simulink model "ev3_final"  (R2018b)
settings: Solver=FixedStepAuto  StartTime=0.0  StopTime=10.0  RelTol=1e-3  EnableMultiTasking=on
libraries: legoev3lib x9, dspstat3 x2
settings Model: ExtModeTrigDuration=2  Creator=chpark  LastModifiedBy=chpark
settings SolverCC: PositivePriorityOrder=on
settings OptimizationCC: EnhancedBackFolding=on  PassReuseOutputArgsAs=Individual arguments  MaxStackSize=64  OptimizeBlockOrder=speed  DifferentSizesBufferReuse=on  OptimizationCustomize=off
settings DebuggingCC: ParameterTunabilityLossMsg=error
settings HardwareCC: ProdBitPerPointer=32  ProdBitPerSizeT=32  ProdBitPerPtrDiffT=32  ProdLargestAtomicInteger=Long  ProdWordSize=32  ProdHWDeviceType=ARM Compatible->ARM 9  UseEmbeddedCoderFeatures=off  UseSimulinkCoderFeatures=off
settings SFSimCC: MATLABDynamicMemAlloc=off
settings RTWCC: SystemTargetFile=ert.tlc  HardwareBoard=LEGO MINDSTORMS EV3  TLCOptions="-aInlineSetEventsForThisBaseRateFcn=TLC_FALSE -aSuppressMultiTaskScheduler=TLC_FALSE  -aRateBasedStepFcn=0"  TemplateMakefile=ert_default_tmf  GenerateReport=on  Toolchain=Sourcery G++ Lite v2009q3  IncludeHyperlinkInReport=on  LaunchReport=on  GenerateTraceInfo=on  GenerateTraceReport=on  GenerateTraceReportSl=on  GenerateTraceReportSf=on  GenerateTraceReportEml=on
settings CodeAppCC: ForceParamTrailComments=on  IgnoreCustomStorageClasses=off  OperatorAnnotations=on  SimulinkDataObjDesc=on  SFDataObjDesc=on  InsertBlockDesc=on
settings ERTTargetCC: SupportContinuousTime=on  SupportNonInlinedSFcns=on  SupportVariableSizeSignals=on

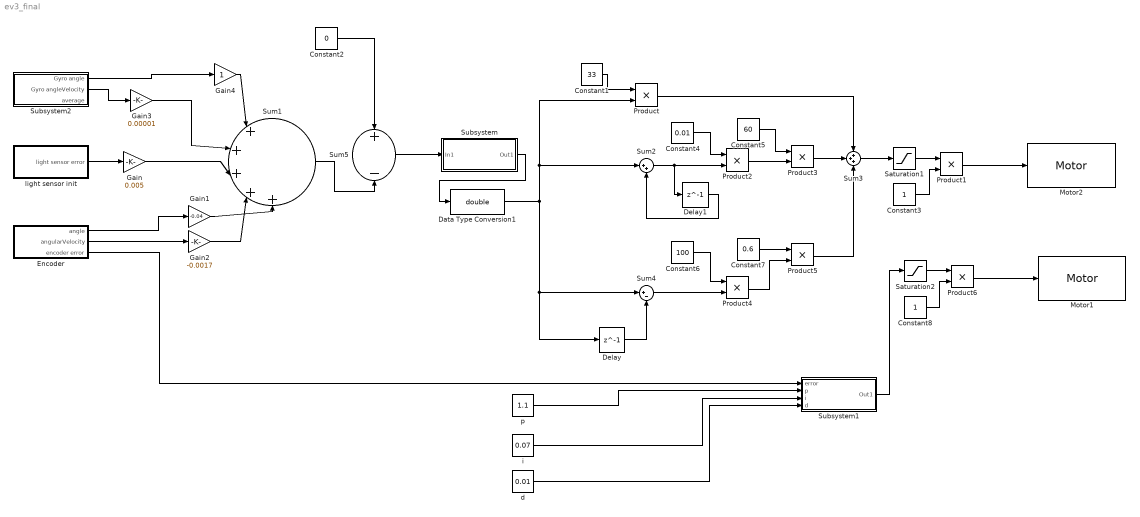
== system ev3_final ==
  Constant1 : Constant  Value=33
  Constant2 : Constant  Value=0
  Constant3 : Constant
  Constant4 : Constant  Value=0.01
  Constant5 : Constant  Value=60
  Constant6 : Constant  Value=100
  Constant7 : Constant  Value=0.6
  Constant8 : Constant
  Data Type Conversion1 : DataTypeConversion  OutDataTypeStr=double
  Delay : Delay  DelayLength=1  InitialCondition=0
  Delay1 : Delay  DelayLength=1  InitialCondition=0
  Encoder : Subsystem
  Gain : Gain  Gain=0.005
  Gain1 : Gain  Gain=-0.04
  Gain2 : Gain  Gain=-0.0017
  Gain3 : Gain  Gain=0.00001
  Gain4 : Gain
  Motor1 : legoev3lib/Motor  sportNumber=D  sstopAction=Brake
  Motor2 : legoev3lib/Motor  sportNumber=A  sstopAction=Brake
  Product{,1..6} (7 alike) : Product
  Saturation1 : Saturate  UpperLimit=100  LowerLimit=-100
  Saturation2 : Saturate  UpperLimit=100  LowerLimit=-100
  Subsystem : Subsystem
  Subsystem1 : Subsystem
  Subsystem2 : Subsystem
  Sum1 : Sum  Inputs=|+++++
  Sum2 : Sum  Inputs=|++
  Sum3 : Sum  Inputs=+++
  Sum4 : Sum  Inputs=|+-
  Sum5 : Sum  Inputs=+-
  d : Constant  Value=0.01
  i : Constant  Value=0.07
  light sensor init : Subsystem
  p : Constant  Value=1.1
  wires:
  Product/1 -> Sum3/1
  Delay1/1 -> Sum2/2
  Subsystem/1(Out1) -> Data Type Conversion1/1
  Saturation1/1 -> Product1/1
  Product2/1 -> Product3/2
  Product1/1 -> Motor2/1
  Product4/1 -> Product5/2
  Constant4/1 -> Product2/1
  Constant1/1 -> Product/1
  Delay/1 -> Sum4/2
  Sum4/1 -> Product4/2
  Constant7/1 -> Product5/1
  Product3/1 -> Sum3/2
  Constant5/1 -> Product3/1
  Sum2/1 -> Product2/2, Delay1/1
  Constant6/1 -> Product4/1
  Constant3/1 -> Product1/2
  Product5/1 -> Sum3/3
  Sum3/1 -> Saturation1/1
  Data Type Conversion1/1 -> Product/2, Sum2/1, Delay/1, Sum4/1
  Encoder/1(angle) -> Gain1/1
  Encoder/2(angularVelocity) -> Gain2/1
  light sensor init/1(light sensor error) -> Gain/1
  Gain/1 -> Sum1/3
  Gain3/1 -> Sum1/2
  Gain4/1 -> Sum1/1
  Sum1/1 -> Sum5/2
  Constant2/1 -> Sum5/1
  Sum5/1 -> Subsystem/1(In1)
  Gain1/1 -> Sum1/5
  Gain2/1 -> Sum1/4
  Subsystem2/1(Gyro angle) -> Gain4/1
  Subsystem2/2(Gyro angleVelocity) -> Gain3/1
  Encoder/3(encoder error) -> Subsystem1/1(error)
  Product6/1 -> Motor1/1
  Constant8/1 -> Product6/2
  Saturation2/1 -> Product6/1
  Subsystem1/1(Out1) -> Saturation2/1
  p/1 -> Subsystem1/2(p)
  i/1 -> Subsystem1/3(i)
  d/1 -> Subsystem1/4(d)

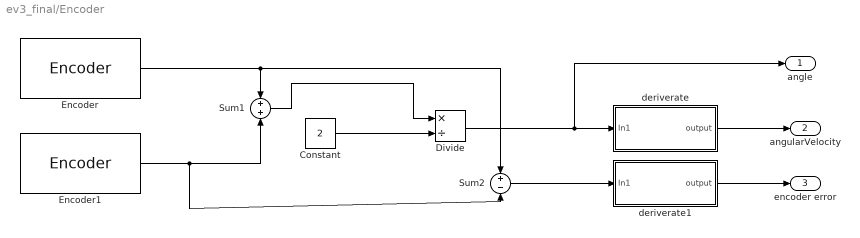
== system ev3_final/Encoder ==
  Constant : Constant  Value=2
  Divide : Product  Inputs=*/
  Encoder : legoev3lib/Encoder  portNumber=A  opMode=Reset by external signal  sampleTime=0.01
      settings: SourceProductName=Simulink Support Package for LEGO MINDSTORMS EV3 Hardware  SourceProductBaseCode=LEGOEV3
  Encoder1 : legoev3lib/Encoder  portNumber=D  opMode=Reset by external signal  sampleTime=0.01
      settings: SourceProductName=Simulink Support Package for LEGO MINDSTORMS EV3 Hardware  SourceProductBaseCode=LEGOEV3
  Sum1 : Sum
  Sum2 : Sum  Inputs=+-
  deriverate : Subsystem
  deriverate1 : Subsystem
  angle : Outport
  angularVelocity : Outport  Port=2
  encoder error : Outport  Port=3
  wires:
  Encoder/1 -> Sum2/1, Sum1/1
  Encoder1/1 -> Sum2/2, Sum1/2
  Constant/1 -> Divide/2
  Sum1/1 -> Divide/1
  Divide/1 -> deriverate/1(In1), angle/1
  deriverate/1(output) -> angularVelocity/1
  Sum2/1 -> deriverate1/1(In1)
  deriverate1/1(output) -> encoder error/1

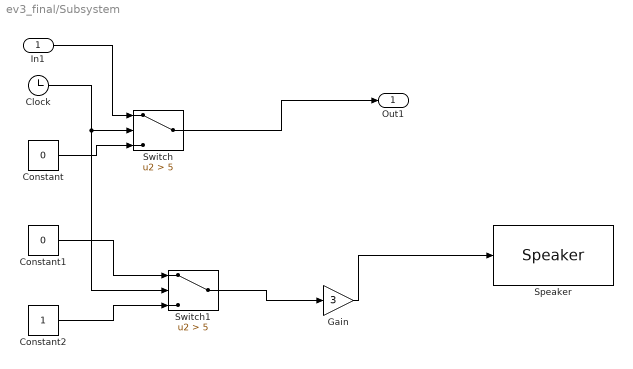
== system ev3_final/Subsystem ==
  In1 : Inport
  Clock : Clock
  Constant : Constant  Value=0
  Constant1 : Constant  Value=0
  Constant2 : Constant
  Gain : Gain  Gain=3
  Speaker : legoev3lib/Speaker  sinputMode=Volume only  sspeakerFreq=100  sspeakerVolume=50  sspeakerDuration=100
      settings: SourceProductName=Simulink Support Package for LEGO MINDSTORMS EV3 Hardware  SourceProductBaseCode=LEGOEV3
  Switch : Switch  Criteria=u2 > Threshold  Threshold=5
  Switch1 : Switch  Criteria=u2 > Threshold  Threshold=5
  Out1 : Outport
  wires:
  Clock/1 -> Switch1/2, Switch/2
  In1/1 -> Switch/1
  Constant/1 -> Switch/3
  Constant1/1 -> Switch1/1
  Constant2/1 -> Switch1/3
  Gain/1 -> Speaker/1
  Switch1/1 -> Gain/1
  Switch/1 -> Out1/1

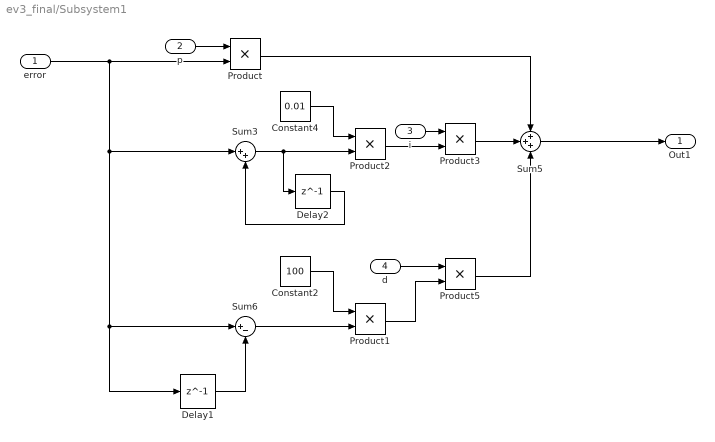
== system ev3_final/Subsystem1 ==
  error : Inport
  p : Inport  Port=2
  i : Inport  Port=3
  d : Inport  Port=4
  Constant2 : Constant  Value=100
  Constant4 : Constant  Value=0.01
  Delay1 : Delay  DelayLength=1  InitialCondition=0
  Delay2 : Delay  DelayLength=1  InitialCondition=0
  Product{,1..3,5} (5 alike) : Product
  Sum3 : Sum  Inputs=|++
  Sum5 : Sum  Inputs=+++
  Sum6 : Sum  Inputs=|+-
  Out1 : Outport
  wires:
  Product2/1 -> Product3/2
  Constant4/1 -> Product2/1
  Sum6/1 -> Product1/2
  Sum3/1 -> Product2/2, Delay2/1
  Product5/1 -> Sum5/3
  Constant2/1 -> Product1/1
  Product3/1 -> Sum5/2
  d/1 -> Product5/1
  Delay1/1 -> Sum6/2
  Product1/1 -> Product5/2
  Delay2/1 -> Sum3/2
  Product/1 -> Sum5/1
  error/1 -> Delay1/1, Sum6/1, Sum3/1, Product/2
  Sum5/1 -> Out1/1
  p/1 -> Product/1
  i/1 -> Product3/1

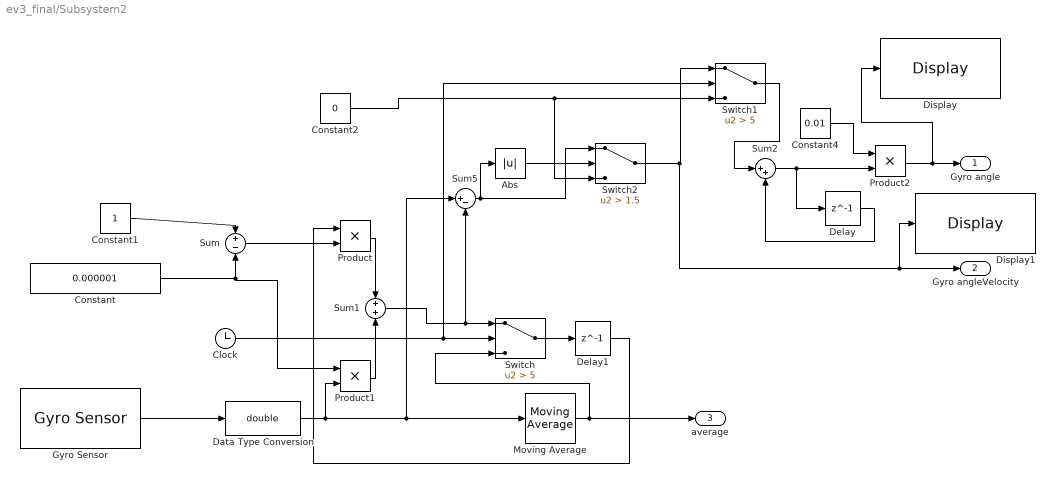
== system ev3_final/Subsystem2 ==
  Abs : Abs
  Clock : Clock
  Constant : Constant  Value=0.000001
  Constant1 : Constant
  Constant2 : Constant  Value=0
  Constant4 : Constant  Value=0.01
  Data Type Conversion : DataTypeConversion  OutDataTypeStr=double
  Delay : Delay  DelayLength=1  InitialCondition=0
  Delay1 : Delay  DelayLength=1  InitialCondition=0
  Display : legoev3lib/Display  slcdLine=3  slcdFormat=Decimal
      settings: SourceProductName=Simulink Support Package for LEGO MINDSTORMS EV3 Hardware  SourceProductBaseCode=LEGOEV3
  Display1 : legoev3lib/Display  slcdLine=5  slcdFormat=Decimal
      settings: SourceProductName=Simulink Support Package for LEGO MINDSTORMS EV3 Hardware  SourceProductBaseCode=LEGOEV3
  Gyro Sensor : legoev3lib/Gyro Sensor  portNumber=1  sampleTime=0.01
      settings: SourceProductName=Simulink Support Package for LEGO MINDSTORMS EV3 Hardware  SourceProductBaseCode=LEGOEV3
  Moving Average : dspstat3/Moving Average  Method=Sliding window  ForgettingFactorPort=off  SpecifyWindowLength=on  WindowLength=300  ForgettingFactor=0.9  SimulateUsing=Code generation
  Product : Product
  Product1 : Product
  Product2 : Product
  Sum : Sum  Inputs=+-
  Sum1 : Sum
  Sum2 : Sum  Inputs=|++
  Sum5 : Sum  Inputs=|+-
  Switch : Switch  Criteria=u2 > Threshold  Threshold=5
  Switch1 : Switch  Criteria=u2 > Threshold  Threshold=5
  Switch2 : Switch  Criteria=u2 > Threshold  Threshold=1.5
  Gyro angle : Outport
  Gyro angleVelocity : Outport  Port=2
  average : Outport  Port=3
  wires:
  Switch/1 -> Delay1/1
  Gyro Sensor/1 -> Data Type Conversion/1
  Moving Average/1 -> average/1, Switch/3
  Data Type Conversion/1 -> Product1/2, Moving Average/1, Sum5/1
  Sum5/1 -> Abs/1, Switch2/1
  Clock/1 -> Switch1/2, Switch/2
  Constant1/1 -> Sum/1
  Constant/1 -> Product1/1, Sum/2
  Sum/1 -> Product/2
  Product/1 -> Sum1/1
  Product1/1 -> Sum1/2
  Sum1/1 -> Sum5/2, Switch/1
  Delay1/1 -> Product/1
  Constant4/1 -> Product2/1
  Delay/1 -> Sum2/2
  Product2/1 -> Display/1, Gyro angle/1
  Sum2/1 -> Delay/1, Product2/2
  Constant2/1 -> Switch2/3, Switch1/3
  Switch1/1 -> Sum2/1
  Abs/1 -> Switch2/2
  Switch2/1 -> Gyro angleVelocity/1, Display1/1, Switch1/1

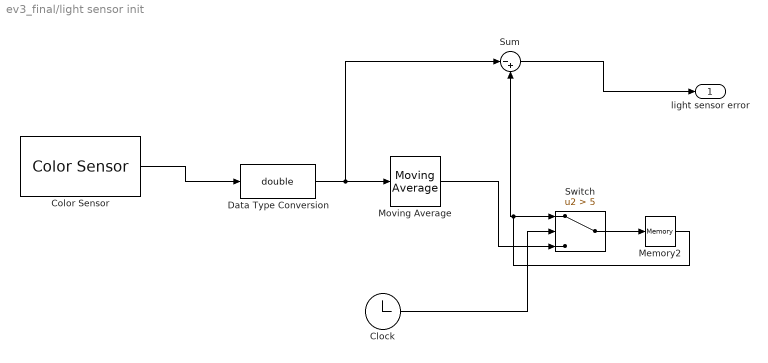
== system ev3_final/light sensor init ==
  Clock : Clock
  Color Sensor : legoev3lib/Color Sensor  portNumber=4  mode=Reflected light intensity  sampleTime=0.01
      settings: SourceProductName=Simulink Support Package for LEGO MINDSTORMS EV3 Hardware  SourceProductBaseCode=LEGOEV3
  Data Type Conversion : DataTypeConversion  OutDataTypeStr=double
  Memory2 : Memory
  Moving Average : dspstat3/Moving Average  Method=Sliding window  ForgettingFactorPort=off  SpecifyWindowLength=on  WindowLength=300  ForgettingFactor=0.9  SimulateUsing=Code generation
  Sum : Sum  Inputs=|-+
  Switch : Switch  Criteria=u2 > Threshold  Threshold=5
  light sensor error : Outport
  wires:
  Switch/1 -> Memory2/1
  Moving Average/1 -> Switch/3
  Color Sensor/1 -> Data Type Conversion/1
  Data Type Conversion/1 -> Sum/1, Moving Average/1
  Clock/1 -> Switch/2
  Memory2/1 -> Sum/2, Switch/1
  Sum/1 -> light sensor error/1

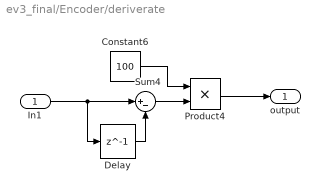
== system ev3_final/Encoder/deriverate ==
  In1 : Inport
  Constant6 : Constant  Value=100
  Delay : Delay  DelayLength=1  InitialCondition=0
  Product4 : Product
  Sum4 : Sum  Inputs=|+-
  output : Outport
  wires:
  Delay/1 -> Sum4/2
  Product4/1 -> output/1
  In1/1 -> Delay/1, Sum4/1
  Sum4/1 -> Product4/2
  Constant6/1 -> Product4/1

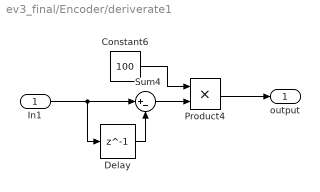
== system ev3_final/Encoder/deriverate1 ==
  In1 : Inport
  Constant6 : Constant  Value=100
  Delay : Delay  DelayLength=1  InitialCondition=0
  Product4 : Product
  Sum4 : Sum  Inputs=|+-
  output : Outport
  wires:
  Delay/1 -> Sum4/2
  Product4/1 -> output/1
  In1/1 -> Delay/1, Sum4/1
  Sum4/1 -> Product4/2
  Constant6/1 -> Product4/1
